simulink model "RoboCarModel"  (R2023a)
settings: Solver=VariableStepAuto  StartTime=0.0  StopTime=10.0  RelTol=1e-3
settings Model: Creator=Franz  LastModifiedBy=Franz
settings DebuggingCC: UnderSpecifiedDimensionMsg=warning

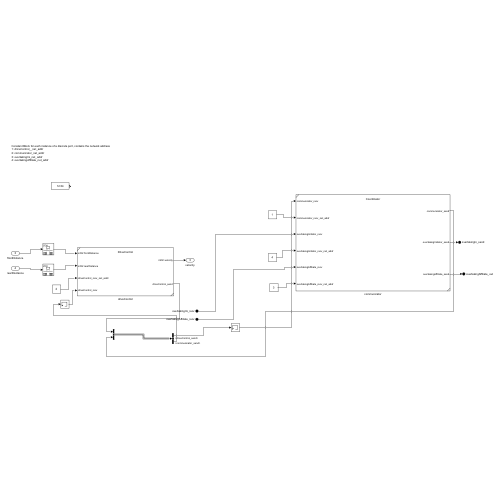
[thumbnail: Simulink's stored preview of the top-level diagram]
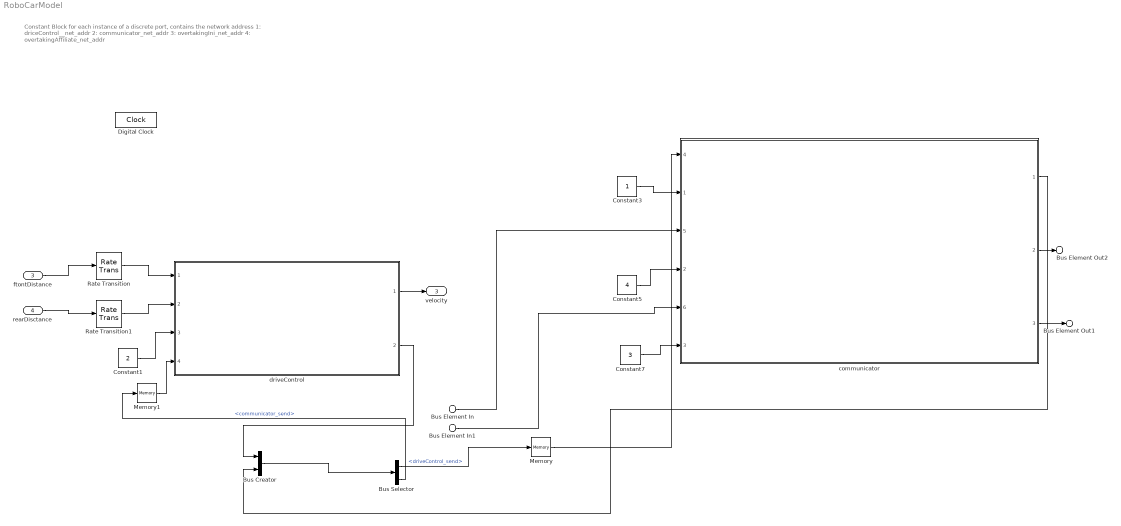
== system RoboCarModel ==
  note: Constant Block for each instance of a discrete port, contains the network address
      | 1: driceControl__net_addr
      | 2: communicator_net_addr
      | 3: overtakingIni_net_addr
      | 4: overtakingAffiliate_net_addr
  Bus Element In : Inport  PortName=overtakingIni_recv
  Bus Element In1 : Inport  Port=2  PortName=overtakingAffiliate_recv
  ftontDistance : Inport  Port=3
  rearDisctance : Inport  Port=4  Interpolate=off
  Bus Creator : BusCreator  Inputs=2
  Bus Selector : BusSelector  OutputSignals=driveControl_send,communicator_send
  Constant1 : Constant  Value=2
  Constant3 : Constant
  Constant5 : Constant  Value=4
  Constant7 : Constant  Value=3
  Digital Clock : DigitalClock
  Memory : Memory
  Memory1 : Memory
  Rate Transition : RateTransition  OutPortSampleTime=30
  Rate Transition1 : RateTransition  OutPortSampleTime=30
  communicator : Subsystem  ReferencedSubsystem=Coordinator
      settings: PortSchema="{\"entries\":[{\"content\":{\"sides\":[{\"content\":{\"connectorIds\":[\"In4\",\"In1\",\"In5\",\"In2\",\"In6\",\"In3\"]},\"type\":\"ConnectorPlacement.EquallySpacedRectSide\",\"uuid\":\"597f2600-0266-49ee-88a2-3e6a618a9f6e\"},{\"content\":{\"connectorIds\":[\"Out1\",\"Out2\",\"Out3\"],\"side\":\"RIGHT\"},\"type\":\"ConnectorPlacement.EquallySpacedRectSide\",\"uuid\":\"8a05e0df-8602-4cac-b3df-55f21ffd748f\"},{\"content\":{\"side\":\"TOP\"},\"type\":\"ConnectorPlacement.EquallySpacedRectSide\",\"uuid\":\"f3d30c22-937d-4096-90b7-da40b4c40188\"}]},\"type\":\"ConnectorPlacement.EquallySpacedConnector\",\"uuid\":\"be54317e-1502-459c-b560-7b4d203f7350\"}],\"packageUris\":[\"http://schema.mathworks.com/mf0/Connector/R2020b\"],\"version\":\"1.0\"}"
  driveControl : Subsystem  ReferencedSubsystem=DriveControl
  Bus Element Out1 : Outport  PortName=overtakingAffiliate_out
  Bus Element Out2 : Outport  Port=2  PortName=overtakingIn_send
  velocity : Outport  Port=3
  wires:
  driveControl/1 -> velocity/1
  Constant1/1 -> driveControl/3
  Constant3/1 -> communicator/1
  Constant5/1 -> communicator/2
  Constant7/1 -> communicator/3
  driveControl/2 -> Bus Creator/1
  Bus Element In/1 -> communicator/5
  communicator/2 -> Bus Element Out2/1
  communicator/3 -> Bus Element Out1/1
  Bus Element In1/1 -> communicator/6
  Bus Creator/1 -> Bus Selector/1
  Bus Selector/1 -> Memory/1  "<driveControl_send>"
  Bus Selector/2 -> Memory1/1  "<communicator_send>"
  Memory/1 -> communicator/4
  communicator/1 -> Bus Creator/2
  Memory1/1 -> driveControl/4
  ftontDistance/1 -> Rate Transition/1
  rearDisctance/1 -> Rate Transition1/1
  Rate Transition/1 -> driveControl/1
  Rate Transition1/1 -> driveControl/2
